simulink model "Motor_Model_lag"  (R2023a)
settings: Solver=ode4  StartTime=0.0  StopTime=3  FixedStep=0.001  RelTol=1e-3
values from neighbouring files (symbols this model uses):
  b = 0.1    [setup_motor_closed_loop.m]
  J = 0.01    [setup_motor_closed_loop.m]
  K = 0.01    [setup_motor_closed_loop.m]
  L = 0.5    [setup_motor_closed_loop.m]
  R = 1.0    (= 1)    [setup_motor_closed_loop.m]
settings Model: Creator=sansh  LastModifiedBy=Fasih
settings SolverCC: AlgebraicLoopSolver=TrustRegion
settings DataIOCC: ReturnWorkspaceOutputs=off
settings DebuggingCC: UnconnectedInputMsg=warning  UnconnectedOutputMsg=warning  UnconnectedLineMsg=warning  ArithmeticOperatorsInVariantConditions=warning
settings ModelReferenceCC: EnableRefExpFcnMdlSchedulingChecks=on
settings SFSimCC: SimUseLocalCustomCode=off  CustomCodeUndefinedFunction=UseInterfaceOnly
settings RTWCC: RTWUseLocalCustomCode=off
settings CodeAppCC: StateflowObjectComments=on

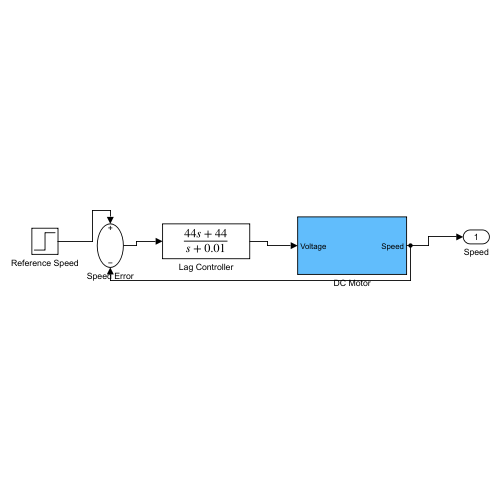
[thumbnail: Simulink's stored preview of the top-level diagram]
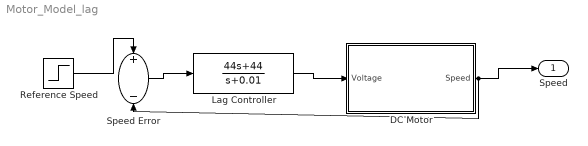
== system Motor_Model_lag ==
  DC Motor : Subsystem
  Lag Controller : TransferFcn  Numerator=[44 44]  Denominator=[1 0.01]
  Reference Speed : Step  Time=0  SampleTime=0
  Speed Error : Sum  Inputs=+-
  Speed : Outport
  wires:
  Reference Speed/1 -> Speed Error/1
  Speed Error/1 -> Lag Controller/1
  Lag Controller/1 -> DC Motor/1(Voltage)
  DC Motor/1(Speed) -> Speed/1, Speed Error/2

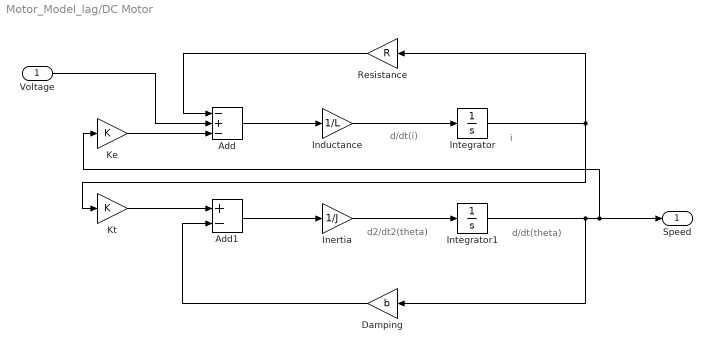
== system Motor_Model_lag/DC Motor ==
  note: i
  note: d/dt(i)
  note: d/dt(theta)
  note: d2/dt2(theta)
  Voltage : Inport
  Add : Sum  Inputs=-+-
  Add1 : Sum  Inputs=+-
  Damping : Gain  Gain=b
  Inductance : Gain  Gain=1/L
  Inertia : Gain  Gain=1/J
  Integrator : Integrator
  Integrator1 : Integrator
  Ke : Gain  Gain=K
  Kt : Gain  Gain=K
  Resistance : Gain  Gain=R
  Speed : Outport
  wires:
  Inductance/1 -> Integrator/1
  Integrator1/1 -> Damping/1, Speed/1, Ke/1
  Inertia/1 -> Integrator1/1
  Integrator/1 -> Resistance/1, Kt/1
  Kt/1 -> Add1/1
  Voltage/1 -> Add/2
  Resistance/1 -> Add/1
  Damping/1 -> Add1/2
  Ke/1 -> Add/3
  Add/1 -> Inductance/1
  Add1/1 -> Inertia/1
